simulink model "vent_run24"  (R2022a)
settings: Solver=FixedStepAuto  StartTime=0.0  StopTime=30.0  FixedStep=0.05  MinStep=0.01  RelTol=1e-3  EnableMultiTasking=on
libraries: mbedblockslib x23, simulink x13, hdlsllib x6, slpidlib x2
(part 3 of 3)

== system vent_run24/Subsystem/System Update and Heirarchy/Update Internal Variables/HMI_CMD1/User_Input/EPAP ==
  note: EPAP
  Action Port : ActionPort  ActionPortLabel=case [ 1 ]:
  Constant : Constant
  Out1 : Outport
  wires:
  Constant/1 -> Out1/1

== system vent_run24/Subsystem/System Update and Heirarchy/Update Internal Variables/HMI_CMD1/User_Input/FiO2 ==
  note: FiO2
  Action Port : ActionPort  ActionPortLabel=case [ 3 ]:
  Constant : Constant  Value=3
  Out1 : Outport
  wires:
  Constant/1 -> Out1/1

== system vent_run24/Subsystem/System Update and Heirarchy/Update Internal Variables/HMI_CMD1/User_Input/IPAP ==
  note: IPAP
  Action Port : ActionPort  ActionPortLabel=case [ 2 ]:
  Constant : Constant  Value=2
  Out1 : Outport
  wires:
  Constant/1 -> Out1/1

== system vent_run24/Subsystem/System Update and Heirarchy/Update Internal Variables/HMI_CMD1/User_Input/Not Recognised ==
  note: Must be within array element range [0-3]
  Action Port : ActionPort  ActionPortLabel=default:
  Constant : Constant  Value=0
  Out1 : Outport
  wires:
  Constant/1 -> Out1/1

== system vent_run24/Subsystem/System Update and Heirarchy/Update Internal Variables/HMI_CMD1/User_Input/Subsystem ==
  note: Update single element of input array
  Value1 : Inport
  Element1 : Inport  Port=2
  Assignment : Assignment  IndexMode=Zero-based  DiagnosticForDimensions=Warning  IndexOptions=Index vector (port)  Indices=0  OutputSizes=1
  Constant5 : Constant  Value=[0,0,0,0]
  Arr1 : Outport
  wires:
  Assignment/1 -> Arr1/1
  Element1/1 -> Assignment/3
  Value1/1 -> Assignment/2
  Constant5/1 -> Assignment/1

== system vent_run24/Subsystem/System Update and Heirarchy/Update Internal Variables/HMI_CMD1/User_Input/TTP ==
  note: Time To Peak
  Action Port : ActionPort  ActionPortLabel=case [ 5 ]:
  Constant : Constant  Value=5
  Out1 : Outport
  wires:
  Constant/1 -> Out1/1

== system vent_run24/Subsystem/System Update and Heirarchy/Update Internal Variables/HMI_CMD1/User_Input/Upper4 ==
  note: Get Upper 4 bits
  u : Inport
  Bit Shift1 : hdlsllib/Logic and Bit Operations/Bit Shift  mode=Shift Right Logical  N=4
  Data Type Conversion1 : DataTypeConversion  OutDataTypeStr=uint8  SaturateOnIntegerOverflow=off  RndMeth=Floor
  Extract Bits3 : simulink/Logic and Bit Operations/Extract Bits  bitsToExtract=Upper half  numBits=8  bitIdxRange=[0 7]  outScalingMode=Preserve fixed-point scaling
  y : Outport
  wires:
  u/1 -> Extract Bits3/1
  Extract Bits3/1 -> Data Type Conversion1/1
  Bit Shift1/1 -> y/1
  Data Type Conversion1/1 -> Bit Shift1/1

== stateflow chart vent_run24/Subsystem/Power Sub-Systems/POWER ==
  note: Add IPAP & EPAP initial values
      | Never to happen again
  state Run % Power Up Sequence
    state Lets_Begin % Power Up
      entry: % none
      HMI_Pwr = 1;
      ALRM_Pwr = 1;
      exit: % none
    state HMI_On % Power HMI
      entry:
      HMI_Pwr = 0; % LED Off
      exit:
    state Alrm_On % Power ALRM
      entry:
      ALRM_Pwr = 0;
      exit:
    (default) -> Lets_Begin % Power Up
    Lets_Begin % Power Up -> HMI_On % Power HMI : after(1,sec)
    HMI_On % Power HMI -> Alrm_On % Power ALRM : after(500,msec)
  note: Was:
      | HMI=1;    --> Off
      | ALRM=1; --> Off
      |
      | 2sec
      |
      | HMI=0     --> On
      |
      | 2sec
      |
      | ALRM=0; --> On
  (default) -> Run % Power Up Sequence
  data: HMI_Pwr output; ALRM_Pwr output

== stateflow chart vent_run24/Subsystem/Sub-Systems Read/HMI_Test_Input/Startup - Motor Test ==
  note: Start - EPAP(6) - IPAP(15) - CPAP Mode - Stop
  state stop_start
    entry:
    output = [17,1];
    exit:
  state EPAP
    entry:
    output = [19,6];
    exit:
  state IPAP
    entry:
    output = [35,15];
    exit:
  state MODE_B
    entry:
    output = [09,1];
    exit:
  state Stop_Mtr
    entry:
    output = [1,1];
    exit:
  note: 0x01 (01) - Stop
      | 0x11 (17) - Start
      | [2nd value ignored]
  note: 0x13 ( 19 ) - EPAP
      | 0x08 (0 8) - Value
  note: 0x23 ( 35 ) - IPAP
      | 0x0F ( 15 ) - Value
  note: 0x09 (09) - CPAP
      | 0x19 (25) - BiPAP
      | [2nd value ignored]
  note: 0x01 (01) - Stop
      | 0x11 (17) - Start
      | [2nd value ignored]
  (default) -> stop_start
  MODE_B -> Stop_Mtr : after(25,sec)
  EPAP -> IPAP : after(1,sec)
  IPAP -> MODE_B : after(2,sec)
  stop_start -> EPAP : after(1,sec)
  data: output output uint8

== stateflow chart vent_run24/Subsystem/System Update and Heirarchy/Bootup Values/Init_Vals ==
  state ONCE
    entry:
    nope = 0;
    exit:
  state IPAP
    entry:
    nope = nope + 1;
    output = [35,15];
    exit:
  state EPAP
    entry:
    nope = nope + 1;
    output = [19,5];
    exit:
  state CPAP
    entry:
    nope = nope + 1;
    output = [3,6];
    exit:
  note: Array clears this value
      | Increase the array by one & ignore
  state FiO2
    entry:
    nope = nope + 1;
    output = [51,22];
    exit:
  note: Add state:
      | Initial FiO2 = 22%
      | 0x33 = [51, 22]
  state Default1 % init_vals
    entry:
    nope = nope + 1;
    exit:
  (default) -> ONCE
  ONCE -> IPAP : after(50,msec)
  IPAP -> EPAP : after(50,msec)
  EPAP -> CPAP : after(50,msec)
  CPAP -> FiO2 : after(50,msec)
  FiO2 -> Default1 % init_vals : after(50,msec)
  data: output output uint8; nope output

== stateflow chart vent_run24/Subsystem/Motor Controller/Motor_Ctrl1 ==
  state SHUTDOWN % Blower Off
    state Stop_1 % I2C to Anal.
      entry: mtr = 0;
      exit:
    state Stop_2 % Motor Brake
      entry:
      mtr_brk = 0; % Enable
      exit:
    state Stop_3 % Motor Disable
      entry:
      mtr_dis = 0; % Disable
      exit:
    state Stop_4 % Main Power
      entry:
      mtr_pwr = 0; % OFF
      exit:
    (default) -> Stop_1 % I2C to Anal.
    Stop_1 % I2C to Anal. -> Stop_2 % Motor Brake : after(1,sec)
    Stop_2 % Motor Brake -> Stop_3 % Motor Disable : after(1,sec)
    Stop_3 % Motor Disable -> Stop_4 % Main Power : after(1,sec)
  state STARTUP % Blower Start
    state Start_1 % Main Power
      entry:
      mtr_pwr = 1; % ON
      exit:
    state Start_2 % Motor Brake
      entry:
      mtr_brk = 1; % Disable
      mtr_dis = 1; % Enabled
      exit:
    (default) -> Start_1 % Main Power
    Start_1 % Main Power -> Start_2 % Motor Brake : after(1,sec)
  state Run_Mtr %
    entry: mtr =1;
    exit:
  note: 1. Power - On
      | 2. Brake - Off
      | 3. Disable - Off
      | 4. Voltage Output
  note: BRAKE PIN:
      | Enabled = <0.8V or Gnd
      | Deactivated = >2.4V or Not wired
  note: DISABLE PIN:
      | Disable = <0.8V or Gnd
      | Enable = >2.4V or Not wired
  note: Continuously check for Start/Stop
  (default) -> STARTUP % Blower Start
  STARTUP % Blower Start -> Run_Mtr % : after(2,sec)
  Run_Mtr % -> SHUTDOWN % Blower Off [order 1] : after(180,sec)
  Run_Mtr % -> (junction 37) [order 2] : after(1,sec)
  (junction 37) -> SHUTDOWN % Blower Off [order 2] : [power == 0]
  (junction 37) -> Run_Mtr % [order 1] : [power==1]
  (junction 44) -> STARTUP % Blower Start [order 1] : [power==1]
  (junction 44) -> SHUTDOWN % Blower Off [order 2] : [power==0]
  SHUTDOWN % Blower Off -> (junction 44) : after(4, sec)
  data: mtr output; mtr_brk output; mtr_pwr output; power input; mtr_dis output

== stateflow chart vent_run24/Subsystem/Sub-Systems Read/HMI_Test_Input/Startup - Ex_Valve Test ==
  note: EPAP(6) - IPAP(15) - CPAP Mode - Start - Stop
  state EPAP1
    entry:
    output = [19,6];
    exit:
  state EPAP
    entry:
    output = [35,15];
    exit:
  state MODE_B1
    entry:
    output = [09,1];
    exit:
  state stop_start
    entry:
    output = [17,1];
    exit:
  state Stop_Mtr
    entry:
    output = [1,1];
    exit:
  note: 0x01 (01) - Stop
      | 0x11 (17) - Start
      | [2nd value ignored]
  note: 0x13 ( 19 ) - EPAP
      | 0x08 (0 8) - Value
  note: 0x23 ( 35 ) - IPAP
      | 0x0F ( 15 ) - Value
  note: 0x09 (09) - CPAP
      | 0x19 (25) - BiPAP
      | [2nd value ignored]
  note: 0x01 (01) - Stop
      | 0x11 (17) - Start
      | [2nd value ignored]
  (default) -> EPAP1
  stop_start -> Stop_Mtr : after(35,sec)
  EPAP -> MODE_B1 : after(1,sec)
  MODE_B1 -> stop_start : after(2,sec)
  EPAP1 -> EPAP : after(1,sec)
  data: output output uint8

== stateflow chart vent_run24/Subsystem/Sub-Systems Read/HMI_Test_Input/Startup - Mode Test ==
  note: Start - EPAP(4) - IPAP(16) - BiPAP Mode - CPAP Mode - Stop
  state stop_start
    entry:
    output = [17,1];
    exit:
  state EPAP
    entry:
    output = [19,4];
    exit:
  state IPAP
    entry:
    output = [35,16];
    exit:
  state MODE_B
    entry:
    output = [25,1];
    exit:
  state MODE_C
    entry:
    output = [9,0];
    exit:
  state Stop_Mtr
    entry:
    output = [1,1];
    exit:
  note: 0x01 (01) - Stop
      | 0x11 (17) - Start
      | [2nd value ignored]
  note: 0x13 ( 19 ) - EPAP
      | 0x08 (0 8) - Value
  note: 0x23 ( 35 ) - IPAP
      | 0x0F ( 15 ) - Value
  note: 0x09 (09) - CPAP
      | 0x19 (25) - BiPAP
      | [2nd value ignored]
  note: 0x09 (09) - CPAP
      | 0x19 (25) - BiPAP
      | [2nd value ignored]
  note: 0x01 (01) - Stop
      | 0x11 (17) - Start
      | [2nd value ignored]
  (default) -> stop_start
  EPAP -> IPAP : after(1,sec)
  MODE_B -> MODE_C : after(16,sec)
  MODE_C -> Stop_Mtr : after(10,sec)
  IPAP -> MODE_B : after(2,sec)
  stop_start -> EPAP : after(1,sec)
  data: output output uint8

== stateflow chart vent_run24/Subsystem/Motor Controller/Motor_Ctrl ==
  state SHUTDOWN % Blower Off
    state Stop_1 % I2C to Anal.
      entry: mtr = 0;
      exit:
    state Stop_2 % Motor Brake
      entry:
      mtr_brk = 0; % Enable
      exit:
    state Stop_3 % Motor Disable
      entry:
      mtr_dis = 0; % Disable
      exit:
    state Stop_4 % Main Power
      entry:
      mtr_pwr = 0; % OFF
      exit:
    (default) -> Stop_1 % I2C to Anal.
    Stop_1 % I2C to Anal. -> Stop_2 % Motor Brake : after(2,sec)
    Stop_2 % Motor Brake -> Stop_3 % Motor Disable : after(500,msec)
    Stop_3 % Motor Disable -> Stop_4 % Main Power : after(1,sec)
  state STARTUP % Blower Start
    state Start_1 % Main Power
      entry:
      mtr_pwr = 0; % ON
      mtr_brk = 0; % Enabled
      mtr_dis = 0; % Disabled
      exit:
    (default) -> STARTUP.Start_1 % Main Power
  state Start_Mtr % Blower On
    state Start_1 % Main Power
      entry:
      mtr_pwr = 1; % ON
      exit:
    state Start_2 % Motor Brake
      entry:
      mtr_brk = 1; % Disable
      mtr_dis = 1; % Enabled
      exit:
    (default) -> Start_Mtr.Start_1 % Main Power
    Start_Mtr.Start_1 % Main Power -> Start_2 % Motor Brake : after(1,sec)
  state Run_Mtr % Continuous
    entry: mtr =1; % I2C output
    exit:
    note: Continuously Run the
        | Motor until Stop bit set
  note: Stop Motor after 3min
  note: Wait for Start
  note: POWER PIN:
      | Disable = <0.8V or Gnd
      | Enable = >30V or Not wired
  note: BRAKE PIN:
      | Enabled = <0.8V or Gnd
      | Deactivated = >2.4V or Not wired
  note: DISABLE PIN:
      | Disable = <0.8V or Gnd
      | Enable = >2.4V or Not wired
  note: Continuously check
      | for Start/Stop
  note: 1. Power - On
      | 2. Brake - Off
      | 3. Disable - Off
      | 4. Voltage Output
  (default) -> STARTUP % Blower Start
  Run_Mtr % Continuous -> SHUTDOWN % Blower Off [order 1] : after(180,sec)
  STARTUP % Blower Start -> (junction 53) : after(100,msec)
  (junction 53) -> Start_Mtr % Blower On [order 1] : [power == 1]
  (junction 53) -> STARTUP % Blower Start [order 2] : [power == 0]
  Start_Mtr % Blower On -> Run_Mtr % Continuous : after(2,sec)
  Run_Mtr % Continuous -> (junction 37) [order 2] : after(500,msec)
  (junction 37) -> SHUTDOWN % Blower Off [order 2] : [power == 0]
  (junction 37) -> Run_Mtr % Continuous [order 1] : [power==1]
  SHUTDOWN % Blower Off -> STARTUP % Blower Start : after(4, sec)
  data: mtr output; mtr_brk output; mtr_pwr output; power input; mtr_dis output

== stateflow chart vent_run24/Subsystem/Motor Controller/LED ==
  note: TEST:
      | Routine Checks
  state Run % Parent
    state Check % Check Sub-Systems
      entry:
      LED = 0; % LED Off
      exit:
    state LED % Child
      entry: % none
      LED = 1; % LED On
      exit: % none
    (default) -> LED % Child
    LED % Child -> Check % Check Sub-Systems : after(1,sec)
    Check % Check Sub-Systems -> LED % Child : after(3,sec)
  note: Check Input
      | Power present?
  (default) -> Run % Parent
  data: LED output

== stateflow chart vent_run24/Subsystem/Synchronise_Timing/Alt_Inputs ==
  note: Mode(0) = CPAP
      | Mode(1) = BiPAP
  note: Change back to:
      | [Mode == 1]
  state BiPAP
    state IPAP_out
      entry:
      during:
      xPAP = IPAP;
      exhale = 85; % Open?
      exit:
    note: Inhale:
        | IPAP(15)
        | after(2.6,sec)
    state EPAP_out
      entry:
      during:
      xPAP = EPAP;
      exhale = 15; % Closed?
      exit:
    note: Exhale:
        | EPAP(5)
        | after(1.4,sec)
    (default) -> IPAP_out
    BiPAP.EPAP_out -> IPAP_out : after(2.6,sec)
    IPAP_out -> BiPAP.EPAP_out : after(1.4,sec)
  state CPAP
    state IPAP_in
      entry:
      during:
      xPAP = CPAP; % (fix)
      exhale = 85; % Open?
      exit:
    note: Continuous
        | Pressure
        | Maintained
    state EPAP_out
      entry:
      during:
      exhale = 15; % Closed?
      exit:
    note: Exhale:
        | EPAP(5)
        | after(1.4,sec)
    (default) -> IPAP_in
    CPAP.EPAP_out -> IPAP_in : after(2.6,sec)
    IPAP_in -> CPAP.EPAP_out : after(1.4,sec)
  note: Swap these back:
      | <-------->
  (default) -> (junction 23)
  (junction 23) -> BiPAP [order 1] : [Mode == 1]
  (junction 23) -> CPAP [order 2]
  (junction 54) -> (junction 23)
  BiPAP -> (junction 54) : [Mode == 0]
  CPAP -> (junction 54) : [Mode == 1]
  data: Mode input; CPAP input; exhale output; EPAP input; IPAP input; xPAP output
